simulink model "PredatorPrey"  (R2024b)
settings: Solver=VariableStepAuto  StartTime=0.0  StopTime=100.0  RelTol=1e-3
settings Model: Creator=max  LastModifiedBy=max

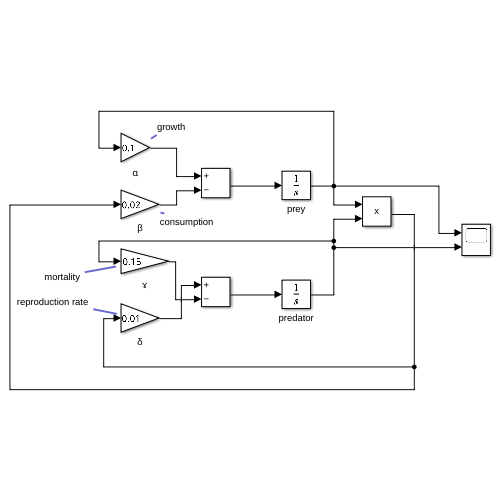
[thumbnail: Simulink's stored preview of the top-level diagram]
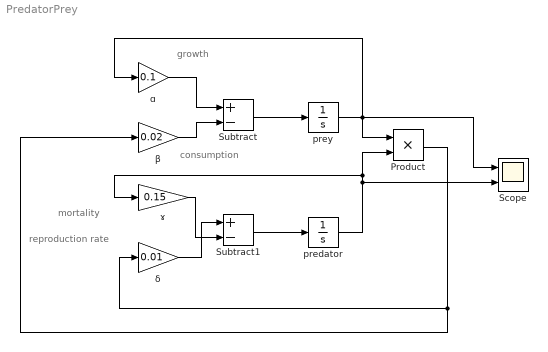
== system PredatorPrey ==
  note: reproduction rate
  note: mortality
  note: consumption
  note: growth
  Product : Product
  Scope : Scope  NumInputPorts=2
  Subtract : Sum  Inputs=+-
  Subtract1 : Sum  Inputs=+-
  predator : Integrator  InitialCondition=5
  prey : Integrator  InitialCondition=10
  ɑ : Gain  Gain=0.1
  ɤ : Gain  Gain=0.15
  β : Gain  Gain=0.02
  δ : Gain  Gain=0.01
  wires:
  ɑ/1 -> Subtract/1
  β/1 -> Subtract/2
  Subtract/1 -> prey/1
  prey/1 -> Scope/1, Product/1, ɑ/1
  Subtract1/1 -> predator/1
  predator/1 -> Product/2, ɤ/1, Scope/2
  Product/1 -> β/1, δ/1
  δ/1 -> Subtract1/1
  ɤ/1 -> Subtract1/2
